simulink model "MpcSim"  (R2024a)
settings: Solver=VariableStepAuto  StartTime=0.0  StopTime=5  RelTol=1e-3
values from neighbouring files (symbols this model uses):
  A = [0 1;-0.00012 -65.45]    [MPC.m]
  B = [0 ; 44.05]    [MPC.m]
  C = [1 0]    [MPC.m]
  D = 0    [MPC.m]
  K = place(A,B,p)    [MPC.m]
  Kr = (1/stepin.Peak)    [MPC.m]
libraries: mpclib x1
settings Model: Creator=mingyangpan  LastModifiedBy=mingyangpan

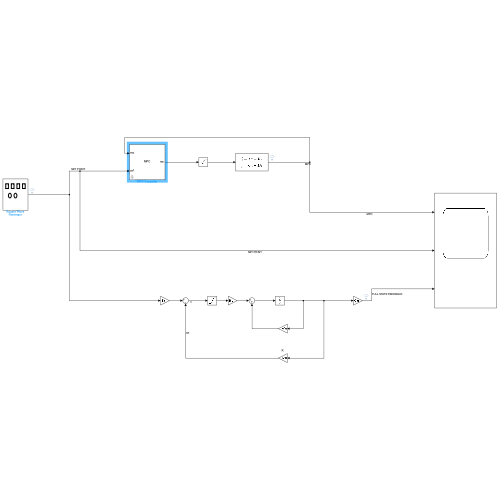
[thumbnail: Simulink's stored preview of the top-level diagram]
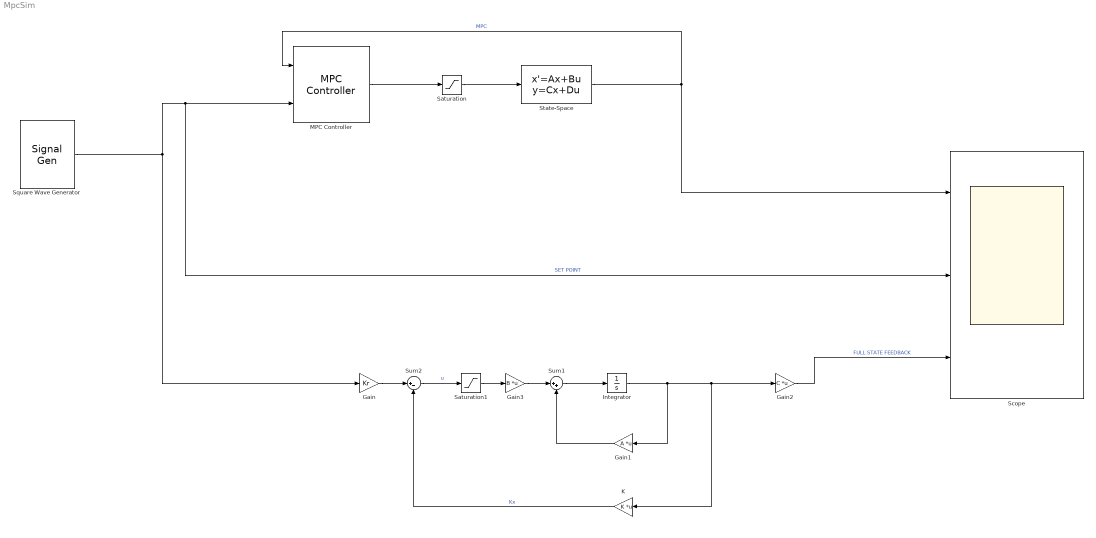
== system MpcSim ==
  Gain : Gain  Gain=Kr
  Gain1 : Gain  Gain=A  Multiplication=Matrix(K*u)
  Gain2 : Gain  Gain=C  Multiplication=Matrix(K*u)
  Gain3 : Gain  Gain=B  Multiplication=Matrix(K*u)
  Integrator : Integrator
  K : Gain  Gain=K  Multiplication=Matrix(K*u)
  MPC Controller : mpclib/MPC Controller  SCDEnableBlockLinearizationSpecification=on  mpcobj=mpc1  is_multiple=0  enable_value=0  return_u0=off  updateMPCinCallerWorkspace=on  md_inport=off  mv_inport=off  uref_inport=off  return_cost=off  return_mvseq=off  return_qpstatus=off  return_xseq=off  return_state=off  return_ovseq=off  state_inport=off  umin_inport=off  umax_inport=off  ymin_inport=off  ymax_inport=off  cc_inport=off  ywt_inport=off  uwt_inport=off  duwt_inport=off  rhoeps_inport=off  pm_inport=off  MaximumP=10  HorizonChoice=FixedHorizon  n_ts=0.01  n_p=6  n_mv=1  n_md=0  n_ud=0  n_mo=1  n_uo=0  BlockDataType=double  SampleTimeInherited=off  switch_inport=off
  Saturation : Saturate  UpperLimit=300  LowerLimit=-300
  Saturation1 : Saturate  UpperLimit=300  LowerLimit=-300
  Scope : Scope  NumInputPorts=3
  Square Wave Generator : SignalGenerator  WaveForm=sawtooth  Amplitude=10  Frequency=0.4
  State-Space : StateSpace  A=A  B=B  C=C  D=D  InitialCondition=0
  Sum1 : Sum  Inputs=|++
  Sum2 : Sum  Inputs=|+-
  wires:
  Square Wave Generator/1 -> Gain/1, MPC Controller/2, Scope/2  "SET POINT"
  State-Space/1 -> MPC Controller/1, Scope/1  "MPC"
  Gain2/1 -> Scope/3  "FULL STATE FEEDBACK"
  K/1 -> Sum2/2  "Kx"
  Gain/1 -> Sum2/1
  Gain3/1 -> Sum1/1
  Sum1/1 -> Integrator/1
  Gain1/1 -> Sum1/2
  Saturation1/1 -> Gain3/1
  MPC Controller/1 -> Saturation/1
  Saturation/1 -> State-Space/1
  Sum2/1 -> Saturation1/1  "u"
  Integrator/1 -> K/1, Gain2/1, Gain1/1
